simulink model "model_T_PSH_IEEE39"  (R2020b)
settings: Solver=ode3  StartTime=0.0  StopTime=300  FixedStep=Ts  RelTol=1e-3
PostLoadFcn:
  | IEEE39BusLineLength;
  | vNomHV = 345E3;fNom=60;load('Dynamicload.mat');
InitFcn:
  | IEEE39BusLineLength;
  | vNomHV = 345E3;fNom=60;load('Dynamicload.mat');
values from neighbouring files (symbols this model uses):
  At = 1.48    [MAIN_T_PSH_IEEE39.m]
  Dturb = 0.3    [MAIN_T_PSH_IEEE39.m]
  fix_mode = 1    [MAIN_T_PSH_IEEE39.m]
  Gmax = 1    [MAIN_T_PSH_IEEE39.m]
  Gmin = 0    [MAIN_T_PSH_IEEE39.m]
  Hdam = 1    [MAIN_T_PSH_IEEE39.m]
  Kd = 1    [MAIN_T_PSH_IEEE39.m]    (also in plots_T_PSH_IEEE39.m)
  max_delay_gen2pump = 20    [MAIN_T_PSH_IEEE39.m]
  max_delay_pump2hsc = 30    [MAIN_T_PSH_IEEE39.m]
  pgen_pump = Kd*Pref    (= 0.9)    [MAIN_T_PSH_IEEE39.m]
  pgen_turb = (1-Kd)*Pref    (= 0)    [MAIN_T_PSH_IEEE39.m]
  pgen_turb_gen2pump = (1-kd_gen2pump)*Pref    (= 0)    [MAIN_T_PSH_IEEE39.m]
  pgen_turb_hsc2gen = (1-kd_hsc2gen)*Pref    (= 0.36)    [MAIN_T_PSH_IEEE39.m]
  pgen_turb_pump2hsc = (1-kd_pump2hsc)*Pref    (= 0.36)    [MAIN_T_PSH_IEEE39.m]
  Pref = 0.9    [MAIN_T_PSH_IEEE39.m]    (also in MAIN_VS_PSH.m = 1)
  qNL = 0.1    [MAIN_T_PSH_IEEE39.m]
  R = 0.04    [MAIN_T_PSH_IEEE39.m]
  r = 0.31    [MAIN_T_PSH_IEEE39.m]
  Rp = 0.05    [IEEE39BusLineLength.m]
  Sn = 320E6    (= 320000000)    [MAIN_T_PSH_IEEE39.m]
  t_gen2pump = 10    [MAIN_T_PSH_IEEE39.m]
  t_hsc2gen = 150    [MAIN_T_PSH_IEEE39.m]
  t_pump2hsc = 35    [MAIN_T_PSH_IEEE39.m]
  t_sw_off = 220    [MAIN_FS_PSH_IEEE39.m]    (also in MAIN_T_PSH_IEEE39.m; MAIN_VS_PSH.m = 45)
  t_sw_on = 130    [MAIN_FS_PSH_IEEE39.m]    (also in MAIN_T_PSH_IEEE39.m; MAIN_VS_PSH.m = 35)
  Tf = 0.05    [MAIN_T_PSH_IEEE39.m]
  Tg = 0.5    [MAIN_T_PSH_IEEE39.m]
  TL_10_11_len = 14    [IEEE39BusLineLength.m]
  TL_10_13_len = 14    [IEEE39BusLineLength.m]
  TL_13_14_len = 32    [IEEE39BusLineLength.m]
  TL_14_15_len = 70    [IEEE39BusLineLength.m]
  TL_15_16_len = 31.5    [IEEE39BusLineLength.m]
  TL_16_17_len = 26    [IEEE39BusLineLength.m]
  TL_16_19_len = 61    [IEEE39BusLineLength.m]
  TL_16_21_len = 46    [IEEE39BusLineLength.m]
  TL_16_24_len = 15    [IEEE39BusLineLength.m]
  TL_17_18_len = 26    [IEEE39BusLineLength.m]
  TL_17_27_len = 59    [IEEE39BusLineLength.m]
  TL_1_2_len = 134    [IEEE39BusLineLength.m]
  TL_1_39_len = 105    [IEEE39BusLineLength.m]
  TL_21_22_len = 47    [IEEE39BusLineLength.m]
  TL_22_23_len = 33    [IEEE39BusLineLength.m]
  TL_24_23_len = 88    [IEEE39BusLineLength.m]
  TL_25_26_len = 101    [IEEE39BusLineLength.m]
  TL_26_27_len = 46.5    [IEEE39BusLineLength.m]
  TL_26_28_len = 151    [IEEE39BusLineLength.m]
  TL_26_29_len = 200    [IEEE39BusLineLength.m]
  TL_28_29_len = 48    [IEEE39BusLineLength.m]
  TL_2_25_len = 28    [IEEE39BusLineLength.m]
  TL_2_2_len = 49    [IEEE39BusLineLength.m]
  TL_3_18_len = 42    [IEEE39BusLineLength.m]
  TL_3_4_len = 53    [IEEE39BusLineLength.m]
  TL_4_14_len = 33    [IEEE39BusLineLength.m]
  TL_4_5_len = 32.5    [IEEE39BusLineLength.m]
  TL_5_6_len = 14    [IEEE39BusLineLength.m]
  TL_5_8_len = 32    [IEEE39BusLineLength.m]
  TL_6_11_len = 26.5    [IEEE39BusLineLength.m]
  TL_6_7_len = 25.5    [IEEE39BusLineLength.m]
  TL_7_8_len = 15    [IEEE39BusLineLength.m]
  TL_8_9_len = 93    [IEEE39BusLineLength.m]
  TL_9_39_len = 136    [IEEE39BusLineLength.m]
  Tr = 6.88    [MAIN_T_PSH_IEEE39.m]
  Ts = 25e-6    (= 2.5e-05)    [MAIN_FS_PSH_IEEE39.m]    (also in MAIN_T_PSH_IEEE39.m; MAIN_VS_PSH.m = 1e-07)
  Velm = 0.05    [MAIN_T_PSH_IEEE39.m]
  Vn = 18000    [MAIN_T_PSH_IEEE39.m]
undefined symbols (not defined in the file or in its folder): D1, Delta, load15, load16, load18, load20, load21, load23, load24, load25, load26, load27, load28, load29, load3, load39, load4, load7, load8
libraries: powerlib x216, sps_avr x10, simulink_extras x7, powerlib_meascontrol x5, simulink x1
(part 3 of 9)

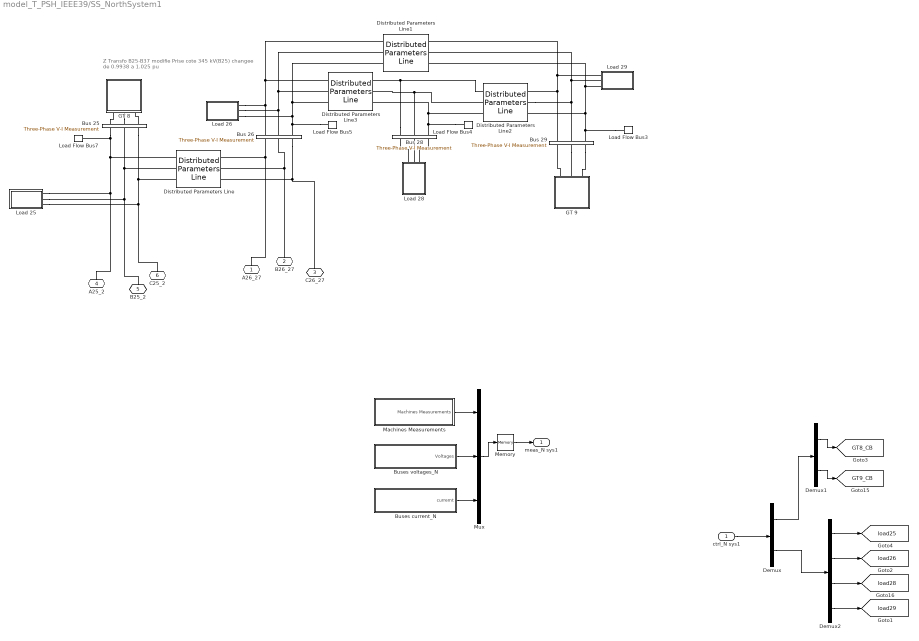
== system model_T_PSH_IEEE39/SS_NorthSystem1 ==
  note: Z Transfo B25-B37 modifie
      | Prise cote 345 kV(B25)  changee de 0.9938 a 1.025 pu
  ctrl_N sys1 : Inport
  Bus 25 : powerlib/Measurements/Three-Phase V-I Measurement  VoltageMeasurement=phase-to-ground  SetLabelV=on  LabelV=V_bus_25  Vpu=off  VpuLL=off  CurrentMeasurement=yes  SetLabelI=on  LabelI=I_bus_25  Ipu=off  Pbase=100e6  Vbase=230e3  OutputType=Complex  PhasorSimulation=off  PSBequivalent=0
  Bus 26 : powerlib/Measurements/Three-Phase V-I Measurement  VoltageMeasurement=phase-to-ground  SetLabelV=on  LabelV=V_bus_26  Vpu=off  VpuLL=off  CurrentMeasurement=yes  SetLabelI=on  LabelI=I_bus_26  Ipu=off  Pbase=100e6  Vbase=230e3  OutputType=Complex  PhasorSimulation=off  PSBequivalent=0
  Bus 28 : powerlib/Measurements/Three-Phase V-I Measurement  VoltageMeasurement=phase-to-ground  SetLabelV=on  LabelV=V_bus_28  Vpu=off  VpuLL=off  CurrentMeasurement=yes  SetLabelI=on  LabelI=I_bus_28  Ipu=off  Pbase=100e6  Vbase=230e3  OutputType=Complex  PhasorSimulation=off  PSBequivalent=0
  Bus 29 : powerlib/Measurements/Three-Phase V-I Measurement  VoltageMeasurement=phase-to-ground  SetLabelV=on  LabelV=V_bus_29  Vpu=off  VpuLL=off  CurrentMeasurement=yes  SetLabelI=on  LabelI=I_bus_29  Ipu=off  Pbase=100e6  Vbase=230e3  OutputType=Complex  PhasorSimulation=off  PSBequivalent=0
  Buses current_N : Subsystem
  Buses voltages_N : Subsystem
  Demux : Demux  Outputs=[2 8]
  Demux1 : Demux  Outputs=2
  Demux2 : Demux  Outputs=[2 2 2 2]
  Distributed Parameters Line : powerlib/Elements/Distributed Parameters Line  Phases=3  Length=TL_25_26_len  Frequency=fNom  Resistance=[3.809 15.235]/TL_25_26_len  Inductance=[0.102 0.306]/TL_25_26_len  Capacitance=[1.143e-6 0.52e-6]/TL_25_26_len  x1=[-0.0004 2.15508784572076e-09 0 0;-0.000375 1.92090052524088e-09 0 0;-0.00035 1.68654257926951e-09 153396.032735497 -197826.091714931;-0.000325 1.45203482483449e-09 155253.647750331 -196371.603628866;-0.0003 1.21739809227051e-09 157097.472238479 -194899.672681526;-0.000275 9.82653223368868e-10 158927.34242079 -193410.42961833;-0.00025 7.47821069526123e-10 160743.095757613 -191904.006722456;-0.000225 5.12922489892006e-10 162544.570963239 -190380.537803097;-0.0002 2.77978349516567e-10 164331.608020222 -188840.158183571;-0.000175 4.30095174968261e-11 166104.048193599 -187283.004689302;-0.00015 -1.91963134876944e-10 167861.734044986 -185709.215635667;-0.000125 -4.26918735975125e-10 169604.509446561 -184118.930815711;-0.0001 -6.6183641568269e-10 171332.219594936 -182512.291487725;-7.5e-05 -8.96695307253009e-10 173044.711024908 -180889.440362705;-5e-05 -1.13147454916136e-09 174741.831623084 -179250.521591671;-2.5e-05 -1.36615328695795e-09 176423.4306414 -177595.680752865]  x2=[-0.0004 1.15306357981996e-08 0 0;-0.000375 1.12211974601005e-08 0 0;-0.00035 1.09107623903608e-08 127977.656266889 -213139.767078873;-0.000325 1.05993581636186e-08 129980.725946247 -211924.157549488;-0.0003 1.02870124405976e-08 131972.249985964 -210689.723691062;-0.000275 9.9737529656512e-09 133952.051487361 -209436.575153149;-0.00025 9.65960756429711e-09 135919.95459302 -208164.823247647;-0.000225 9.34460414074635e-09 137875.78450241 -206874.580938915;-0.0002 9.02877067542436e-09 139819.367487409 -205565.962833734;-0.000175 8.71213522248572e-09 141750.530907737 -204239.085171132;-0.00015 8.39472590732218e-09 143669.103226295 -202894.065812053;-0.000125 8.07657092406441e-09 145574.914024395 -201531.024228895;-0.0001 7.75769853307762e-09 147467.794016903 -200150.081494893;-7.5e-05 7.43813705845132e-09 149347.575067272 -198751.360273364;-5e-05 7.11791488548344e-09 151214.090202481 -197334.984806816;-2.5e-05 6.79706045815894e-09 153067.173627864 -195901.080905906]  x3=[-0.0004 8.25439448304128e-11 0 0;-0.000375 8.29000743756992e-11 0 0;-0.00035 8.3248840257043e-11 8.84459606303463 -75.3299783173848;-0.000325 8.3590211495042e-11 9.55411396660103 -75.2432799021666;-0.0003 8.3924157767129e-11 10.2627832185221 -75.1498979437632;-0.000275 8.42506494102653e-11 10.9705408706972 -75.0498407369003;-0.00025 8.45696574235752e-11 11.6773240559994 -74.9431171692373;-0.000225 8.48811534709225e-11 12.3830699938595 -74.8297367205788;-0.0002 8.51851098834271e-11 13.0877159958426 -74.7097094620317;-0.000175 8.54814996619231e-11 13.7911994712165 -74.5830460551111;-0.00015 8.57702964793565e-11 14.4934579325112 -74.4497577507933;-0.000125 8.60514746831241e-11 15.1944290010697 -74.309856388516;-0.0001 8.63250092973521e-11 15.8940504125887 -74.1633543951273;-7.5e-05 8.65908760251144e-11 16.592260022649 -74.0102647837813;-5e-05 8.6849051250591e-11 17.2889958122359 -73.8506011527823;-2.5e-05 8.70995120411657e-11 17.9841958932482 -73.6843776843774]  x4=[-0.0004 -5.99583731942907e-11 0 0;-0.000375 -6.10035620981299e-11 0 0;-0.00035 -6.20433323128549e-11 835.985708047 -1347.6015887162;-0.000325 -6.30775914800631e-11 848.649206987729 -1339.66287497358;-0.0003 -6.4106247730875e-11 861.237323998919 -1331.60516462833;-0.000275 -6.51292096940947e-11 873.748940931231 -1323.42917341288;-0.00025 -6.61463865043258e-11 886.182946430505 -1315.13562756606;-0.000225 -6.71576878100425e-11 898.538236036478 -1306.72526376854;-0.0002 -6.81630237816154e-11 910.813712280888 -1298.19882907748;-0.000175 -6.91623051192906e-11 923.008284784957 -1289.55708086011;-0.00015 -7.01554430611218e-11 935.120870356245 -1280.80078672647;-0.000125 -7.11423493908544e-11 947.150393084865 -1271.93072446123;-0.0001 -7.21229364457619e-11 959.095784439053 -1262.94768195461;-7.5e-05 -7.30971171244322e-11 970.955983360079 -1253.85245713239;-5e-05 -7.40648048945047e-11 982.729936356497 -1244.64585788503;-2.5e-05 -7.50259138003563e-11 994.416597597726 -1235.3287019959]  x5=0.000398898483326272  V1=ones(3,3)  V2=ones(3,3)  I1=ones(3,3)  I2=ones(3,3)  nHarmo=1  Measurements=None  Decoupling=off  VsMag0=0  VrMag0=0  VsAngle0=0  VrAngle0=0  IsMag0=0  IrMag0=0  IsAngle0=0  IrAngle0=0
  Distributed Parameters Line1 : powerlib/Elements/Distributed Parameters Line  Phases=3  Length=TL_26_29_len  Frequency=fNom  Resistance=[6.784 27.138]/TL_26_29_len  Inductance=[0.197 0.592]/TL_26_29_len  Capacitance=[2.293e-6 1.043e-6]/TL_26_29_len  x1=[-0.0008 1.63239641230318e-08 0 0;-0.000775 1.60341439993032e-08 0 0;-0.00075 1.57428996301936e-08 0 0;-0.000725 1.54502568857118e-08 0 0;-0.0007 1.51562417600785e-08 0 0;-0.000675 1.48608803694171e-08 100969.382894424 -227182.870356359;-0.00065 1.45641989494343e-08 103106.003318764 -226221.181775521;-0.000625 1.4266223853089e-08 105233.465271721 -225239.398921284;-0.0006 1.39669815482524e-08 107351.579779821 -224237.609001278;-0.000575 1.36664986153562e-08 109460.158699888 -223215.901000277;-0.00055 1.3364801745032e-08 111559.014735749 -222174.365672292;-0.000525 1.30619177357401e-08 113647.961454876 -221113.095532513;-0.0005 1.27578734913896e-08 115726.813304943 -220032.184849091;-0.000475 1.24526960189483e-08 117795.385630308 -218931.729634762;-0.00045 1.21464124260438e-08 119853.494688416 -217811.827638322;-0.000425 1.18390499185559e-08 121900.957666121 -216672.578335942;-0.0004 1.15306357981996e-08 123937.592695923 -215514.082922331;-0.000375 1.12211974601005e-08 125963.218872122 -214336.444301751;-0.00035 1.09107623903608e-08 127977.656266889 -213139.767078873;-0.000325 1.05993581636186e-08 129980.725946247 -211924.157549488;-0.0003 1.02870124405976e-08 131972.249985964 -210689.723691062;-0.000275 9.9737529656512e-09 133952.051487361 -209436.575153149;-0.00025 9.65960756429711e-09 135919.95459302 -208164.823247647;-0.000225 9.34460414074635e-09 137875.78450241 -206874.580938915;-0.0002 9.02877067542436e-09 139819.367487409 -205565.962833734;-0.000175 8.71213522248572e-09 141750.530907737 -204239.085171132;-0.00015 8.39472590732218e-09 143669.103226295 -202894.065812053;-0.000125 8.07657092406441e-09 145574.914024395 -201531.024228895;-0.0001 7.75769853307762e-09 147467.794016903 -200150.081494893;-7.5e-05 7.43813705845132e-09 149347.575067272 -198751.360273364;-5e-05 7.11791488548344e-09 151214.090202481 -197334.984806816;-2.5e-05 6.79706045815894e-09 153067.173627864 -195901.080905906]  x2=[-0.0008 7.4949439139317e-09 0 0;-0.000775 7.04361368272204e-09 0 0;-0.00075 6.59165779701819e-09 0 0;-0.000725 6.13911640215519e-09 0 0;-0.0007 5.68602969547636e-09 0 0;-0.000675 5.23243792276278e-09 122729.749227375 -209956.770964221;-0.00065 4.77838137465842e-09 124703.052917168 -208790.76354746;-0.000625 4.32390038309129e-09 126665.279760754 -207606.210127831;-0.0006 3.8690353176909e-09 128616.255461801 -206403.215924219;-0.000575 3.41382658220244e-09 130555.806723366 -205181.887793524;-0.00055 2.95831461089787e-09 132483.76126329 -203942.334221173;-0.000525 2.50253986498429e-09 134399.947829505 -202684.665311482;-0.0005 2.04654282900995e-09 136304.19621524 -201408.992777874;-0.000475 1.59036400726823e-09 138196.337274142 -200115.429932961;-0.00045 1.13404392019974e-09 140076.202935303 -198804.091678474;-0.000425 6.77623100793107e-10 141943.626218184 -197475.094495059;-0.0004 2.21142090984572e-10 143798.441247452 -196128.556431929;-0.000375 -2.3535856194315e-10 145640.483267711 -194764.597096383;-0.00035 -6.91838308962533e-10 147469.588658139 -193383.337643174;-0.000325 -1.14825660290304e-09 149285.594947018 -191984.900763754;-0.0003 -1.60457290205273e-09 151088.34082617 -190569.410675371;-0.000275 -2.06074667375947e-09 152877.666165282 -189136.993110042;-0.00025 -2.5167373980312e-09 154653.412026131 -187687.775303375;-0.000225 -2.97250457113521e-09 156415.420676702 -186221.885983276;-0.0002 -3.42800770919589e-09 158163.535605198 -184739.45535851;-0.000175 -3.88320635179075e-09 159897.601533945 -183240.615107137;-0.00015 -4.33806006554436e-09 161617.46443318 -181725.498364815;-0.000125 -4.79252844771985e-09 163322.971534736 -180194.239712973;-0.0001 -5.24657112980773e-09 165013.971345609 -178646.975166859;-7.5e-05 -5.70014778111166e-09 166690.313661421 -177083.842163455;-5e-05 -6.15321811233084e-09 168351.849579753 -175504.979549274;-2.5e-05 -6.60574187913877e-09 169998.431513378 -173910.527568023]  x3=[-0.0008 9.79065124798276e-11 0 0;-0.000775 9.71058710325094e-11 0 0;-0.00075 9.62966040802502e-11 0 0;-0.000725 9.547878350682e-11 0 0;-0.0007 9.46524819557708e-11 0 0;-0.000675 9.38177728239841e-11 496.962430278397 -1074.70240898626;-0.00065 9.29747302551514e-11 507.06899703311 -1069.97100289853;-0.000625 9.21234291331883e-11 517.130522987582 -1065.14455579965;-0.0006 9.12639450755826e-11 527.146114418902 -1060.22349640255;-0.000575 9.0396354426678e-11 537.114881684327 -1055.20826182418;-0.00055 8.95207342508924e-11 547.035939300309 -1050.09929754668;-0.000525 8.86371623258728e-11 556.908406021145 -1044.89705737779;-0.0005 8.77457171355865e-11 566.731404917259 -1039.60200341056;-0.000475 8.68464778633496e-11 576.50406345309 -1034.2146059823;-0.00045 8.59395243847938e-11 586.2255135646 -1028.73534363281;-0.000425 8.50249372607713e-11 595.894891736381 -1023.16470306185;-0.0004 8.41027977301985e-11 605.511339078354 -1017.50317908592;-0.000375 8.31731877028404e-11 615.074001402063 -1011.75127459432;-0.00035 8.22361897520349e-11 624.582029296547 -1005.90950050446;-0.000325 8.12918871073578e-11 634.034578203794 -999.978375716497;-0.0003 8.03403636472298e-11 643.430808493752 -993.958427067227;-0.000275 7.93817038914667e-11 652.769885538919 -987.850189283298;-0.00025 7.8415992993771e-11 662.050979788471 -981.654204933707;-0.000225 7.74433167341684e-11 671.273266841953 -975.371024381612;-0.0002 7.64637615113885e-11 680.435927522505 -969.001205735437;-0.000175 7.547741433519e-11 689.538147949626 -962.545314799307;-0.00015 7.44843628186322e-11 698.579119611466 -956.003925022783;-0.000125 7.34846951702929e-11 707.558039436649 -949.377617449927;-0.0001 7.24785001864326e-11 716.474109865597 -942.666980667693;-7.5e-05 7.14658672431078e-11 725.326538921381 -935.872610753641;-5e-05 7.04468862882316e-11 734.114540280067 -928.995111222993;-2.5e-05 6.94216478335844e-11 742.837333340562 -922.035092975023]  x4=[-0.0008 -5.17456975158117e-11 0 0;-0.000775 -5.18664554762217e-11 0 0;-0.00075 -5.19826063581593e-11 0 0;-0.000725 -5.20941398444314e-11 0 0;-0.0007 -5.22010460279891e-11 0 0;-0.000675 -5.23033154128068e-11 65.2652956784844 -486.990497559691;-0.00065 -5.24009389147266e-11 69.8520707663282 -486.353768509503;-0.000625 -5.24939078622645e-11 74.4326411893549 -485.67383870545;-0.0006 -5.2582213997381e-11 79.0066000748141 -484.950768542828;-0.000575 -5.26658494762146e-11 83.5735411372306 -484.18462224891;-0.00055 -5.27448068697785e-11 88.1330587144927 -483.37546787724;-0.000525 -5.28190791646204e-11 92.6847478038855 -482.523377301587;-0.0005 -5.28886597634458e-11 97.2282040980659 -481.628426209564;-0.000475 -5.29535424857034e-11 101.763024020975 -480.690694095901;-0.00045 -5.30137215681347e-11 106.288804763687 -479.710264255387;-0.000425 -5.30691916652857e-11 110.805144320187 -478.687223775469;-0.0004 -5.31199478499816e-11 115.311641523082 -477.621663528517;-0.000375 -5.31659856137646e-11 119.807896079233 -476.513678163754;-0.00035 -5.32073008672943e-11 124.293508605313 -475.363366098847;-0.000325 -5.3243889940711e-11 128.768080663282 -474.170829511164;-0.0003 -5.32757495839617e-11 133.231214795776 -472.936174328701;-0.000275 -5.33028769670886e-11 137.682514561415 -471.659510220669;-0.00025 -5.33252696804806e-11 142.121584570018 -470.340950587757;-0.000225 -5.33429257350876e-11 146.548030517717 -468.980612552056;-0.0002 -5.33558435625967e-11 150.96145922199 -467.578616946654;-0.000175 -5.33640220155717e-11 155.361478656581 -466.135088304909;-0.00015 -5.33674603675551e-11 159.747697986322 -464.65015484938;-0.000125 -5.33661583131327e-11 164.119727601851 -463.123948480444;-0.0001 -5.33601159679604e-11 168.477179154217 -461.556604764575;-7.5e-05 -5.33493338687543e-11 172.819665589379 -459.948262922304;-5e-05 -5.33338129732427e-11 177.146801182582 -458.299065815853;-2.5e-05 -5.33135546600814e-11 181.458201572624 -456.609159936445]  x5=0.000785783685246773  V1=ones(3,3)  V2=ones(3,3)  I1=ones(3,3)  I2=ones(3,3)  nHarmo=1  Measurements=None  Decoupling=off  VsMag0=0  VrMag0=0  VsAngle0=0  VrAngle0=0  IsMag0=0  IrMag0=0  IsAngle0=0  IrAngle0=0
  Distributed Parameters Line2 : powerlib/Elements/Distributed Parameters Line  Phases=3  Length=TL_28_29_len  Frequency=fNom  Resistance=[1.666 6.665]/TL_28_29_len  Inductance=[0.048 0.143]/TL_28_29_len  Capacitance=[0.555e-6 0.252e-6]/TL_28_29_len  x1=[-0.0002 3.1750500391877e-09 0 0;-0.000175 2.77150324824847e-09 149843.863072972 -194415.031385725;-0.00015 2.36771027636562e-09 151669.487362494 -192994.171302769;-0.000125 1.96370699076569e-09 153481.639491181 -191556.168361607;-0.0001 1.55952927735648e-09 155280.158493202 -190101.150293973;-7.5e-05 1.15521303753951e-09 157064.884613701 -188629.246342986;-5e-05 7.50794185020978e-10 158835.659322983 -187140.587251666;-2.5e-05 3.4630864262177e-10 160592.3253306 -185635.30525132]  x2=[-0.0002 -3.42800770919589e-09 0 0;-0.000175 -3.88320635179075e-09 159897.601533945 -183240.615107137;-0.00015 -4.33806006554436e-09 161617.46443318 -181725.498364815;-0.000125 -4.79252844771985e-09 163322.971534736 -180194.239712973;-0.0001 -5.24657112980773e-09 165013.971345609 -178646.975166859;-7.5e-05 -5.70014778111166e-09 166690.313661421 -177083.842163455;-5e-05 -6.15321811233084e-09 168351.849579753 -175504.979549274;-2.5e-05 -6.60574187913877e-09 169998.431513378 -173910.527568023]  x3=[-0.0002 9.12220327580155e-11 0 0;-0.000175 8.94525553512782e-11 1148.63643378817 -1167.42336332496;-0.00015 8.7675132251351e-11 1159.58791600809 -1156.5460301779;-0.000125 8.58899213392308e-11 1170.43639692447 -1145.56596592518;-0.0001 8.40970811876731e-11 1181.18091291249 -1134.48414587959;-7.5e-05 8.22967710471066e-11 1191.82050958211 -1123.30155439246;-5e-05 8.04891508314874e-11 1202.35424186285 -1112.01918476622;-2.5e-05 7.8674381104095e-11 1212.7811740877 -1100.63803916619]  x4=[-0.0002 -8.91566494686914e-11 0 0;-0.000175 -8.85123249869826e-11 -139.276268828367 -143.621875375111;-0.00015 -8.78601383287813e-11 -137.916534592532 -144.928119877468;-0.000125 -8.72001474250775e-11 -136.544549812647 -146.221491026229;-0.0001 -8.65324109000793e-11 -135.160436356333 -147.50187393669;-7.5e-05 -8.5856988066006e-11 -133.764317168551 -148.769154877837;-5e-05 -8.51739389178189e-11 -132.35631626068 -150.023221282449;-2.5e-05 -8.44833241278928e-11 -130.936558699501 -151.263961757098]  x5=0.000189831504234676  V1=ones(3,3)  V2=ones(3,3)  I1=ones(3,3)  I2=ones(3,3)  nHarmo=1  Measurements=None  Decoupling=off  VsMag0=0  VrMag0=0  VsAngle0=0  VrAngle0=0  IsMag0=0  IrMag0=0  IsAngle0=0  IrAngle0=0
  Distributed Parameters Line3 : powerlib/Elements/Distributed Parameters Line  Phases=3  Length=TL_26_28_len  Frequency=fNom  Resistance=[5.118 20.472]/TL_26_28_len  Inductance=[0.15 0.449]/TL_26_28_len  Capacitance=[1.739e-6 0.791e-6]/TL_26_28_len  x1=[-0.0006 1.39669815482524e-08 0 0;-0.000575 1.36664986153562e-08 0 0;-0.00055 1.3364801745032e-08 0 0;-0.000525 1.30619177357401e-08 113647.961454876 -221113.095532513;-0.0005 1.27578734913896e-08 115726.813304943 -220032.184849091;-0.000475 1.24526960189483e-08 117795.385630308 -218931.729634762;-0.00045 1.21464124260438e-08 119853.494688416 -217811.827638322;-0.000425 1.18390499185559e-08 121900.957666121 -216672.578335942;-0.0004 1.15306357981996e-08 123937.592695923 -215514.082922331;-0.000375 1.12211974601005e-08 125963.218872122 -214336.444301751;-0.00035 1.09107623903608e-08 127977.656266889 -213139.767078873;-0.000325 1.05993581636186e-08 129980.725946247 -211924.157549488;-0.0003 1.02870124405976e-08 131972.249985964 -210689.723691062;-0.000275 9.9737529656512e-09 133952.051487361 -209436.575153149;-0.00025 9.65960756429711e-09 135919.95459302 -208164.823247647;-0.000225 9.34460414074635e-09 137875.78450241 -206874.580938915;-0.0002 9.02877067542436e-09 139819.367487409 -205565.962833734;-0.000175 8.71213522248572e-09 141750.530907737 -204239.085171132;-0.00015 8.39472590732218e-09 143669.103226295 -202894.065812053;-0.000125 8.07657092406441e-09 145574.914024395 -201531.024228895;-0.0001 7.75769853307762e-09 147467.794016903 -200150.081494893;-7.5e-05 7.43813705845132e-09 149347.575067272 -198751.360273364;-5e-05 7.11791488548344e-09 151214.090202481 -197334.984806816;-2.5e-05 6.79706045815894e-09 153067.173627864 -195901.080905906]  x2=[-0.0006 9.57080391977111e-09 0 0;-0.000575 9.17597950541282e-09 0 0;-0.00055 8.78034002749843e-09 0 0;-0.000525 8.38392062901399e-09 122963.444676142 -212439.234421598;-0.0005 7.98675652222261e-09 124960.134331029 -211270.91365782;-0.000475 7.5888829855367e-09 126945.724304252 -210083.826589902;-0.00045 7.19033536038433e-09 128920.03822423 -208878.07866178;-0.000425 6.79114904807001e-09 130882.900720984 -207653.776974958;-0.0004 6.39135950663013e-09 132834.137441718 -206411.030278989;-0.000375 5.99100224768339e-09 134773.575066304 -205149.948961822;-0.00035 5.59011283327644e-09 136701.041322679 -203870.645039991;-0.000325 5.18872687272504e-09 138616.365002144 -202573.232148666;-0.0003 4.78688001945107e-09 140519.375974576 -201257.825531564;-0.000275 4.38460796781555e-09 142409.905203536 -199924.542030704;-0.00025 3.98194644994808e-09 144287.784761288 -198573.500076038;-0.000225 3.57893123257292e-09 146152.847843711 -197204.819674923;-0.0002 3.17559811383193e-09 148004.928785118 -195818.622401467;-0.000175 2.77198292010485e-09 149843.863072972 -194415.031385725;-0.00015 2.36812150282693e-09 151669.487362494 -192994.171302769;-0.000125 1.9640497353044e-09 153481.639491181 -191556.168361607;-0.0001 1.55980350952806e-09 155280.158493202 -190101.150293973;-7.5e-05 1.15541873298505e-09 157064.884613701 -188629.246342986;-5e-05 7.50931325469441e-10 158835.659322983 -187140.587251666;-2.5e-05 3.46377215891538e-10 160592.3253306 -185635.30525132]  x3=[-0.0006 7.83776307884226e-11 0 0;-0.000575 7.76905428056737e-11 0 0;-0.00055 7.69965538996982e-11 0 0;-0.000525 7.62957257146035e-11 476.255843508178 -929.479031527708;-0.0005 7.55881205020014e-11 484.99465118044 -924.94922486051;-0.000475 7.48738011154781e-11 493.690378823496 -920.33725885501;-0.00045 7.41528310050119e-11 502.342254032538 -915.643543172697;-0.000425 7.34252742113368e-11 510.949508297983 -910.868494736536;-0.0004 7.26911953602539e-11 519.51137707374 -906.012537693939;-0.000375 7.19506596568913e-11 528.027099845119 -901.076103379089;-0.00035 7.1203732879912e-11 536.495920196383 -896.059630274624;-0.000325 7.04504813756712e-11 544.917085877943 -890.963563972692;-0.0003 6.96909720523229e-11 553.289848873169 -885.788357135366;-0.000275 6.89252723738767e-11 561.613465464841 -880.534469454443;-0.00025 6.81534503542054e-11 569.887196301205 -875.202367610604;-0.000225 6.73755745510035e-11 578.110306461649 -869.792525231966;-0.0002 6.65917140596977e-11 586.282065521981 -864.30542285201;-0.000175 6.58019385073092e-11 594.401747619311 -858.741547866894;-0.00015 6.5006318046269e-11 602.468631516527 -853.101394492168;-0.000125 6.42049233481869e-11 610.482000666358 -847.385463718864;-0.0001 6.33978255975736e-11 618.441143275022 -841.594263269006;-7.5e-05 6.25850964855182e-11 626.345352365451 -835.728307550501;-5e-05 6.17668082033197e-11 634.193925840091 -829.788117611455;-2.5e-05 6.09430334360746e-11 641.986166543265 -823.774221093884]  x4=[-0.0006 -3.6346145918975e-11 0 0;-0.000575 -3.65386052331257e-11 0 0;-0.00055 -3.67278189770897e-11 0 0;-0.000525 -3.69137703438082e-11 177.577193825909 -604.634149446868;-0.0005 -3.70964428160056e-11 183.267729700518 -602.933692260166;-0.000475 -3.72758201676568e-11 188.941986675702 -601.179679016695;-0.00045 -3.74518864654282e-11 194.599460731148 -599.372265518053;-0.000425 -3.76246260700931e-11 200.239649337299 -597.511612309156;-0.0004 -3.77940236379211e-11 205.862051499989 -595.597884663982;-0.000375 -3.79600641220408e-11 211.466167804951 -593.631252570885;-0.00035 -3.81227327737762e-11 217.051500462169 -591.6118907175;-0.000325 -3.82820151439572e-11 222.617553350103 -589.539978475222;-0.0003 -3.84378970842027e-11 228.163832059751 -587.415699883276;-0.000275 -3.85903647481773e-11 233.689843938569 -585.23924363237;-0.00025 -3.87394045928217e-11 239.195098134231 -583.010803047932;-0.000225 -3.8885003379555e-11 244.679105638226 -580.730576072941;-0.0002 -3.90271481754511e-11 250.141379329299 -578.398765250341;-0.000175 -3.91658263543875e-11 255.581434016718 -576.015577705051;-0.00015 -3.93010255981662e-11 260.99878648337 -573.58122512557;-0.000125 -3.94327338976089e-11 266.392955528685 -571.095923745168;-0.0001 -3.95609395536227e-11 271.76346201138 -568.559894322686;-7.5e-05 -3.96856311782401e-11 277.109828892015 -565.97336212292;-5e-05 -3.980679769563e-11 282.43158127537 -563.336556896615;-2.5e-05 -3.99244283430816e-11 287.72824645263 -560.649712860058]  x5=0.00059595217928958  V1=ones(3,3)  V2=ones(3,3)  I1=ones(3,3)  I2=ones(3,3)  nHarmo=1  Measurements=None  Decoupling=off  VsMag0=0  VrMag0=0  VsAngle0=0  VrAngle0=0  IsMag0=0  IrMag0=0  IsAngle0=0  IrAngle0=0
  GT 8 : Subsystem
  GT 9 : Subsystem
  Load 25 : Subsystem  SystemSampleTime=20e-3
  Load 26 : Subsystem  SystemSampleTime=20e-3
  Load 28 : Subsystem  SystemSampleTime=20e-3
  Load 29 : Subsystem  SystemSampleTime=20e-3
  Load Flow Bus3 : powerlib/Measurements/Load Flow Bus  LConnTagsString=a  Phases=single  Connectors=on one side  ID=Bus-29  Vbase=345e+003  Vref=1  Vangle=0  VLF=1.034  VLFb=1  VLFc=1  angleLF=25.68  angleLFb=0  angleLFc=0
      settings: AttributesFormatString=%<ID>\n%<Vbase>V\n%<VLF>pu\n%<angleLF>deg.
  Load Flow Bus4 : powerlib/Measurements/Load Flow Bus  LConnTagsString=a  Phases=single  Connectors=on one side  ID=Bus-28  Vbase=345e+003  Vref=1  Vangle=0  VLF=1.031  VLFb=1  VLFc=1  angleLF=23.66  angleLFb=0  angleLFc=0
      settings: AttributesFormatString=%<ID>\n%<Vbase>V\n%<VLF>pu\n%<angleLF>deg.
  Load Flow Bus5 : powerlib/Measurements/Load Flow Bus  LConnTagsString=a  Phases=single  Connectors=on one side  ID=Bus-26  Vbase=345e+003  Vref=1  Vangle=0  VLF=1.027  VLFb=1  VLFc=1  angleLF=21.79  angleLFb=0  angleLFc=0
      settings: AttributesFormatString=%<ID>\n%<Vbase>V\n%<VLF>pu\n%<angleLF>deg.
  Load Flow Bus7 : powerlib/Measurements/Load Flow Bus  LConnTagsString=a  Phases=single  Connectors=on one side  ID=Bus-25  Vbase=345e+003  Vref=1  Vangle=0  VLF=1.034  VLFb=1  VLFc=1  angleLF=25.05  angleLFb=0  angleLFc=0
      settings: AttributesFormatString=%<ID>\n%<Vbase>V\n%<VLF>pu\n%<angleLF>deg.
  Machines Measurements : Subsystem
      mask Display: disp('Machines Measurements')
  Memory : Memory
  Mux : Mux  Inputs=3
  A26_27 : PMIOPort  Side=Left
  B26_27 : PMIOPort  Port=2  Side=Left
  C26_27 : PMIOPort  Port=3  Side=Left
  A25_2 : PMIOPort  Port=4  Side=Left
  B25_2 : PMIOPort  Port=5  Side=Left
  C25_2 : PMIOPort  Port=6  Side=Left
  meas_N sys1 : Outport
  tag scope: GT8_CB=global, GT9_CB=global, load25=global, load26=global, load28=global, load29=global
  wires:
  Machines Measurements/1(Machines Measurements) -> Mux/1
  Mux/1 -> Memory/1
  Memory/1 -> meas_N sys1/1
  Buses voltages_N/1(Voltages) -> Mux/2
  Buses current_N/1(curremt) -> Mux/3
  ctrl_N sys1/1 -> Demux/1
  Demux/2 -> Demux2/1
  Demux/1 -> Demux1/1
  Demux1/1 -> [GT8_CB]
  Demux1/2 -> [GT9_CB]
  Demux2/1 -> [load25]
  Demux2/2 -> [load26]
  Demux2/3 -> [load28]
  Demux2/4 -> [load29]
  connections:
  Load Flow Bus3/LConn1 -- Load 29/LConn3 -- Distributed Parameters Line1/RConn3 -- Distributed Parameters Line2/RConn3 -- Bus 29/RConn3
  Load 29/LConn2 -- Distributed Parameters Line2/RConn2 -- Bus 29/RConn2 -- Distributed Parameters Line1/RConn2
  Bus 29/LConn3 -- GT 9/RConn3
  Bus 29/LConn2 -- GT 9/RConn2
  GT 9/RConn1 -- Bus 29/LConn1
  Distributed Parameters Line2/LConn2 -- Bus 28/RConn2 -- Distributed Parameters Line3/RConn2
  Load 28/LConn3 -- Bus 28/LConn3
  Load 28/LConn2 -- Bus 28/LConn2
  Load 28/LConn1 -- Bus 28/LConn1
  Bus 25/RConn3 -- GT 8/RConn3
  GT 8/RConn2 -- Bus 25/RConn2
  GT 8/RConn1 -- Bus 25/RConn1
  C25_2/RConn1 -- Bus 25/LConn3 -- Distributed Parameters Line/LConn3 -- Load 25/LConn3
  Load 25/LConn2 -- Bus 25/LConn2 -- Distributed Parameters Line/LConn2 -- B25_2/RConn1
  Load Flow Bus7/LConn1 -- A25_2/RConn1 -- Load 25/LConn1 -- Distributed Parameters Line/LConn1 -- Bus 25/LConn1
  Load Flow Bus5/LConn1 -- Distributed Parameters Line1/LConn3 -- Distributed Parameters Line3/LConn3 -- Load 26/LConn3 -- Bus 26/RConn3
  A26_27/RConn1 -- Bus 26/LConn1 -- Distributed Parameters Line/RConn1
  B26_27/RConn1 -- Bus 26/LConn2 -- Distributed Parameters Line/RConn2
  Bus 26/LConn3 -- C26_27/RConn1 -- Distributed Parameters Line/RConn3
  Load 26/LConn1 -- Distributed Parameters Line1/LConn1 -- Distributed Parameters Line3/LConn1 -- Bus 26/RConn1
  Load 26/LConn2 -- Distributed Parameters Line1/LConn2 -- Distributed Parameters Line3/LConn2 -- Bus 26/RConn2
  Bus 28/RConn1 -- Distributed Parameters Line3/RConn1 -- Distributed Parameters Line2/LConn1
  Load Flow Bus4/LConn1 -- Distributed Parameters Line3/RConn3 -- Distributed Parameters Line2/LConn3 -- Bus 28/RConn3
  Load 29/LConn1 -- Bus 29/RConn1 -- Distributed Parameters Line2/RConn1 -- Distributed Parameters Line1/RConn1
